simulink model "Digitizing_2PC"  (R2014a)
settings: Solver=FixedStepDiscrete  StartTime=0.0  StopTime=0.0  FixedStep=1  RelTol=1e-3
values from neighbouring files (symbols this model uses):
  inputPulse = inputSequence ( 76*10^6, 1, 0, 0, 300*10^-9)    [generateBus.m]    (also in plotSimulinkOutput_grid.m = inputSequence(76.92307692*10^6, 1, 0,1.5*10^-6); pulseModel.m = [75.76*10^6, 10, 0, 0, 1])
libraries: opticalComponentLibrary x24
settings Model: Creator=Nithya Menon  LastModifiedBy=Nithya Menon

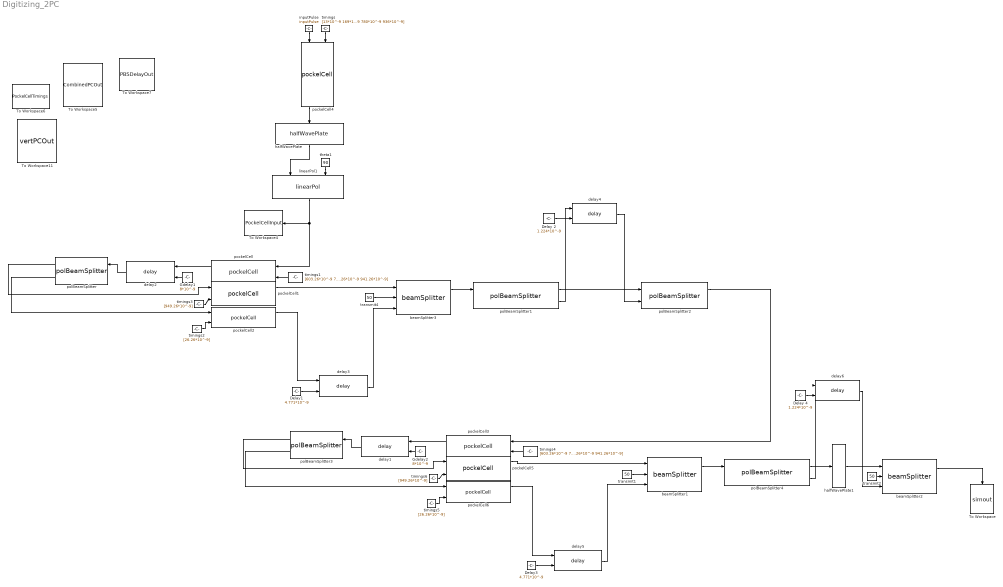
== system Digitizing_2PC ==
  Delay 2 : Constant  Value=1.224*10^-9
  Delay 4 : Constant  Value=1.224*10^-9
  Delay1 : Constant  Value=4.771*10^-9
  Delay3 : Constant  Value=4.771*10^-9
  Gdelay1 : Constant  Value=8*10^-9
  Gdelay2 : Constant  Value=8*10^-9
  To Workspace : ToWorkspace  VariableName=simout  SampleTime=-1
  To Workspace11 : ToWorkspace  VariableName=vertPCOut  SampleTime=-1
  To Workspace4 : ToWorkspace  VariableName=PockelCellInput  SampleTime=-1
  To Workspace5 : ToWorkspace  VariableName=CombinedPCOut  SampleTime=-1
  To Workspace6 : ToWorkspace  VariableName=PockelCellTimings  SampleTime=-1
  To Workspace7 : ToWorkspace  VariableName=PBSDelayOut  SampleTime=-1
  beamSplitter1 : opticalComponentLibrary/beamSplitter
  beamSplitter2 : opticalComponentLibrary/beamSplitter
  beamSplitter3 : opticalComponentLibrary/beamSplitter
  delay{1..6} (6 alike) : opticalComponentLibrary/delay
  halfWavePlate : opticalComponentLibrary/halfWavePlate
  halfWavePlate1 : opticalComponentLibrary/halfWavePlate
  inputPulse : Constant  Value=inputPulse
  linearPol1 : opticalComponentLibrary/linearPol
  pockelCell{,1..6} (7 alike) : opticalComponentLibrary/pockelCell
  polBeamSplitter{,1..4} (5 alike) : opticalComponentLibrary/polBeamSplitter
  theta1 : Constant  Value=90
  timings : Constant  Value="[13*10^-9 169*10^-9 351*10^-9  598*10^-9 780*10^-9 936*10^-9]"
  timings1 : Constant  Value=[603.26*10^-9 785.26*10^-9 941.26*10^-9]
  timings2 : Constant  Value=[26.26*10^-9]
  timings3 : Constant  Value=[949.26*10^-9]
  timings4 : Constant  Value=[603.26*10^-9 785.26*10^-9 941.26*10^-9]
  timings5 : Constant  Value=[26.26*10^-9]
  timings6 : Constant  Value=[949.26*10^-9]
  transmit1 : Constant  Value=50
  transmit2 : Constant  Value=50
  transmit4 : Constant  Value=50
  wires:
  pockelCell/1 -> delay2/1
  Gdelay1/1 -> delay2/2
  delay2/1 -> polBeamSplitter/1
  polBeamSplitter/1 -> pockelCell1/1
  polBeamSplitter/2 -> pockelCell2/1
  Delay1/1 -> delay3/2
  timings1/1 -> pockelCell/2
  timings2/1 -> pockelCell2/2
  timings3/1 -> pockelCell1/2
  beamSplitter3/1 -> polBeamSplitter1/1
  polBeamSplitter1/1 -> polBeamSplitter2/1
  polBeamSplitter1/2 -> delay4/1
  Delay 2/1 -> delay4/2
  delay4/1 -> polBeamSplitter2/2
  linearPol1/1 -> pockelCell/1, To Workspace4/1
  transmit4/1 -> beamSplitter3/2
  pockelCell1/1 -> beamSplitter3/1
  pockelCell4/1 -> halfWavePlate/1
  inputPulse/1 -> pockelCell4/1
  timings/1 -> pockelCell4/2
  halfWavePlate/1 -> linearPol1/1
  theta1/1 -> linearPol1/2
  delay3/1 -> beamSplitter3/3
  pockelCell3/1 -> delay1/1
  Gdelay2/1 -> delay1/2
  delay1/1 -> polBeamSplitter3/1
  polBeamSplitter3/1 -> pockelCell5/1
  polBeamSplitter3/2 -> pockelCell6/1
  Delay3/1 -> delay5/2
  timings4/1 -> pockelCell3/2
  timings5/1 -> pockelCell6/2
  timings6/1 -> pockelCell5/2
  beamSplitter1/1 -> polBeamSplitter4/1
  polBeamSplitter4/2 -> delay6/1
  Delay 4/1 -> delay6/2
  delay6/1 -> beamSplitter2/3
  transmit1/1 -> beamSplitter1/2
  delay5/1 -> beamSplitter1/3
  pockelCell5/1 -> beamSplitter1/1
  pockelCell2/1 -> delay3/1
  pockelCell6/1 -> delay5/1
  polBeamSplitter2/1 -> pockelCell3/1
  polBeamSplitter4/1 -> halfWavePlate1/1
  halfWavePlate1/1 -> beamSplitter2/1
  beamSplitter2/1 -> To Workspace/1
  transmit2/1 -> beamSplitter2/2
